simulink library "write_txt_file"  (R2018b)
settings: Solver=ode45  StartTime=0.0  StopTime=10.0  RelTol=1e-3  EnableMultiTasking=on
settings Model: Creator=lena.frank  LastModifiedBy=drhf
settings DataIOCC: LimitDataPoints=on  SaveFormat=Array  SignalLoggingSaveFormat=ModelDataLogs
settings OptimizationCC: ExpressionDepthLimit=2147483647  LifeSpan=inf
settings DebuggingCC: UnderspecifiedInitializationDetection=Classic  MergeDetectMultiDrivingBlocksExec=none  SolverPrmCheckMsg=warning  FcnCallInpInsideContextMsg=warning  StateNameClashWarn=warning  SFUnexpectedBacktrackingDiag=warning  SFNoUnconditionalDefaultTransitionDiag=warning  SFExecutionAtInitializationDiag=none
settings HardwareCC: ProdBitPerPointer=32  ProdBitPerSizeT=32  ProdBitPerPtrDiffT=32  ProdLargestAtomicFloat=None  ProdIntDivRoundTo=Undefined  ProdEndianess=Unspecified  ProdWordSize=32  ProdHWDeviceType=32-bit Generic
settings ModelReferenceCC: PropagateSignalLabelsOutOfModel=off
settings SFSimCC: SimUseLocalCustomCode=off
settings RTWCC: RTWUseLocalCustomCode=off
settings CodeAppCC: StateflowObjectComments=on
settings GRTTargetCC: TargetLangStandard=C89/C90 (ANSI)  GeneratePreprocessorConditionals=Disable all  CombineOutputUpdateFcns=off  GRTInterface=on
settings ConfigComp: CovMetricSettings=dw  CovHtmlReporting=on  CovSaveCumulativeToWorkspaceVar=on  CovSaveSingleToWorkspaceVar=on  CovExternalEMLEnable=off

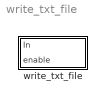
== system write_txt_file ==
  write_txt_file : Subsystem  mask{clear=off, filename='testout.txt'}
      mask prompts: clear "clear existing file"
      mask help:
      | This function writes the input data to a ascii-txt-file, so it can be opened with an usual editor.
      | The data is only written, when the enable signal is 1.
      | It's possible to append data to an existing file or to clear the file before writing.
      |
      | INPUT VECTOR
      |   in         : input data
      |   enable : signal [0,1]
      mask Help: web(fullfile(path_carnot('help'),'write_txt_file.html'),'-helpbrowser')

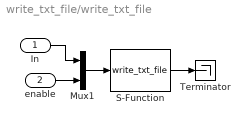
== system write_txt_file/write_txt_file ==
  In : Inport
  enable : Inport  Port=2
  Mux1 : Mux  Inputs=2
  S-Function : S-Function  FunctionName=write_txt_file  Parameters=clear filename  SFunctionDeploymentMode=off  EnableBusSupport=off
  Terminator : Terminator
  wires:
  S-Function/1 -> Terminator/1
  Mux1/1 -> S-Function/1
  In/1 -> Mux1/1
  enable/1 -> Mux1/2
